simulink model "sandbox_6dof"  (R2025b)
settings: Solver=VariableStepAuto  StartTime=0.0  StopTime=10.0  RelTol=1e-3
undefined symbols (not defined in the file): AeroData, Ref_Area, rocket_length
libraries: aerolibconvert2 x3, simulink_extras x2
settings Model: Creator=jonno  LastModifiedBy=jonno

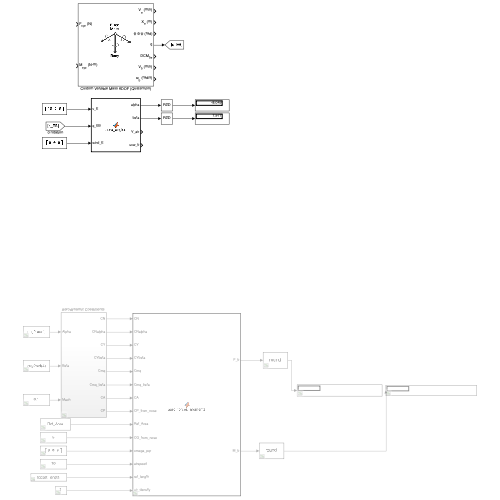
[thumbnail: Simulink's stored preview of the top-level diagram]
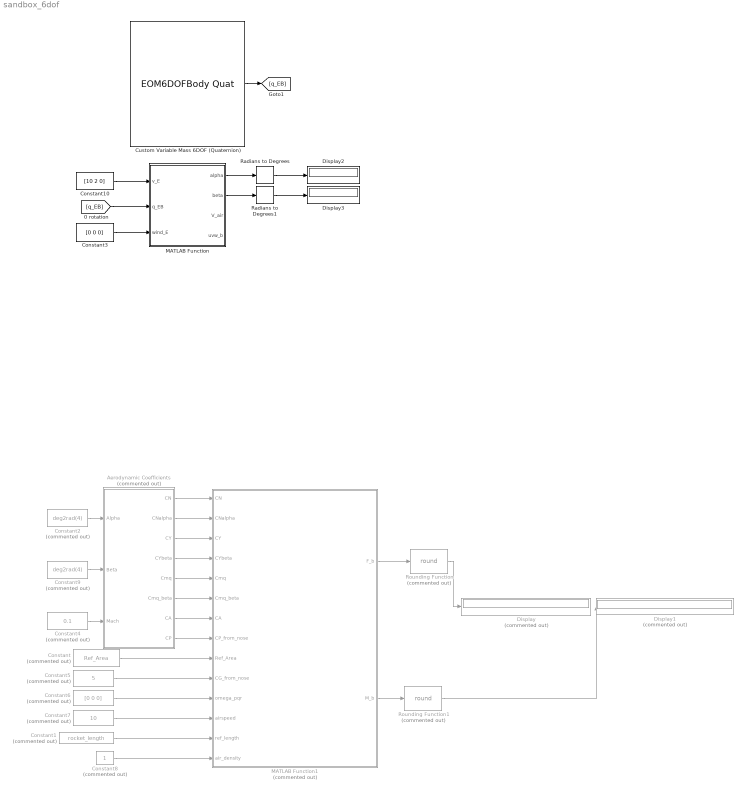
== system sandbox_6dof ==
  "Aerodynamic Coefficients " : Subsystem  Commented=on
  Constant : Constant  Commented=on  Value=Ref_Area  VectorParams1D=off
  Constant1 : Constant  Commented=on  Value=rocket_length
  Constant10 : Constant  Value=[10 2 0]
  Constant2 : Constant  Commented=on  Value=deg2rad(4)
  Constant3 : Constant  Value=[0 0 0]
  Constant4 : Constant  Commented=on  Value=0.1
  Constant5 : Constant  Commented=on  Value=5
  Constant6 : Constant  Commented=on  Value=[0 0 0]
  Constant7 : Constant  Commented=on  Value=10
  Constant8 : Constant  Commented=on
  Constant9 : Constant  Commented=on  Value=deg2rad(4)
  Custom Variable Mass 6DOF (Quaternion) : EOM6DOFBodyQuat  eul_0=[deg2rad(45) deg2rad(0) deg2rad(0)]
  Display : Display  Commented=on
  Display1 : Display  Commented=on
  Display2 : Display
  Display3 : Display
  MATLAB Function : MATLAB Function  TreatAsAtomicUnit=on
  MATLAB Function1 : MATLAB Function  Commented=on  TreatAsAtomicUnit=on
  Radians to Degrees : simulink_extras/Transformations/Radians to Degrees
  Radians to Degrees1 : simulink_extras/Transformations/Radians to Degrees
  Rounding Function : Rounding  Commented=on  Operator=round
  Rounding Function1 : Rounding  Commented=on  Operator=round
  wires:
  Custom Variable Mass 6DOF (Quaternion)/4 -> [q_EB]
  Constant10/1 -> MATLAB Function/1(v_E)
  [q_EB] -> MATLAB Function/2(q_EB)
  MATLAB Function1/1(F_b) -> Rounding Function/1
  Constant5/1 -> MATLAB Function1/10(CG_from_nose)
  Constant6/1 -> MATLAB Function1/11(omega_pqr)
  Constant8/1 -> MATLAB Function1/14(air_density)
  Constant4/1 -> "Aerodynamic Coefficients "/3(Mach)
  Constant2/1 -> "Aerodynamic Coefficients "/1(Alpha)
  "Aerodynamic Coefficients "/4(CYbeta) -> MATLAB Function1/4(CYbeta)
  "Aerodynamic Coefficients "/1(CN) -> MATLAB Function1/1(CN)
  Constant/1 -> MATLAB Function1/9(Ref_Area)
  Constant7/1 -> MATLAB Function1/12(airspeed)
  "Aerodynamic Coefficients "/8(CP) -> MATLAB Function1/8(CP_from_nose)
  "Aerodynamic Coefficients "/6(Cmq_beta) -> MATLAB Function1/6(Cmq_beta)
  "Aerodynamic Coefficients "/5(Cmq) -> MATLAB Function1/5(Cmq)
  Constant9/1 -> "Aerodynamic Coefficients "/2(Beta)
  "Aerodynamic Coefficients "/7(CA) -> MATLAB Function1/7(CA)
  "Aerodynamic Coefficients "/3(CY) -> MATLAB Function1/3(CY)
  "Aerodynamic Coefficients "/2(CNalpha) -> MATLAB Function1/2(CNalpha)
  MATLAB Function1/2(M_b) -> Rounding Function1/1
  Constant1/1 -> MATLAB Function1/13(ref_length)
  Rounding Function1/1 -> Display1/1
  Rounding Function/1 -> Display/1
  MATLAB Function/1(alpha) -> Radians to Degrees/1
  MATLAB Function/2(beta) -> Radians to Degrees1/1
  Constant3/1 -> MATLAB Function/3(wind_E)
  Radians to Degrees/1 -> Display2/1
  Radians to Degrees1/1 -> Display3/1

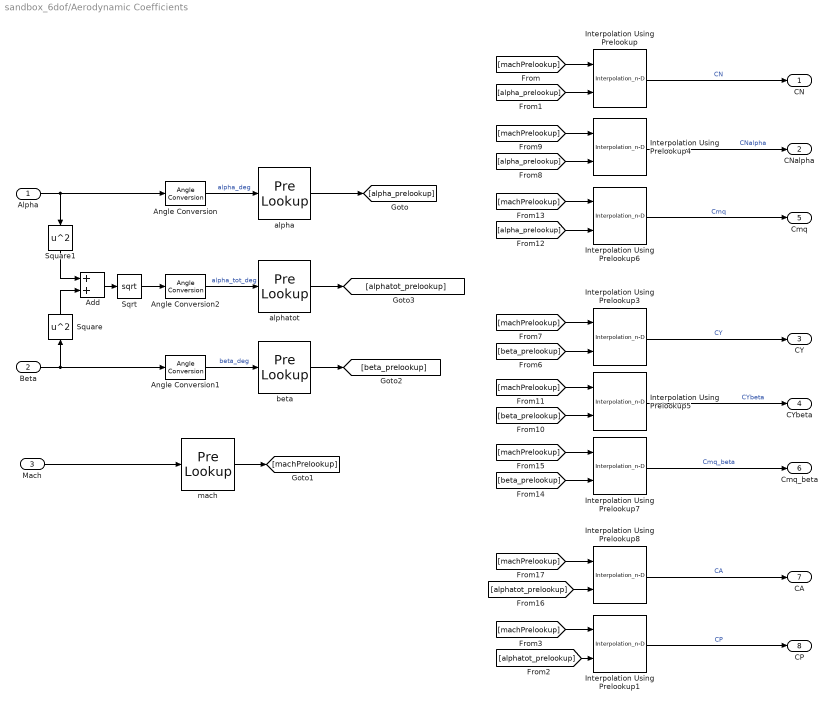
== system sandbox_6dof/Aerodynamic Coefficients  ==
  Alpha : Inport
  Beta : Inport  Port=2
  Mach : Inport  Port=3
  Add : Sum
  Angle Conversion : aerolibconvert2/Angle Conversion  IU=rad  OU=deg
  Angle Conversion1 : aerolibconvert2/Angle Conversion  IU=rad  OU=deg
  Angle Conversion2 : aerolibconvert2/Angle Conversion  IU=rad  OU=deg
  Interpolation Using Prelookup : Interpolation_n-D  Table=AeroData.Tables.CN  RequireIndexFractionAsBus=on  InternalRulePriority=Speed
      settings: InputPortMap=u0,u1
  Interpolation Using Prelookup1 : Interpolation_n-D  Table=AeroData.Tables.CP  RequireIndexFractionAsBus=on  InternalRulePriority=Speed
      settings: InputPortMap=u0,u1
  Interpolation Using Prelookup3 : Interpolation_n-D  Table=AeroData.Tables.CY  RequireIndexFractionAsBus=on  InternalRulePriority=Speed
      settings: InputPortMap=u0,u1
  Interpolation Using Prelookup4 : Interpolation_n-D  Table=AeroData.Tables.CNalpha  RequireIndexFractionAsBus=on  InternalRulePriority=Speed
      settings: InputPortMap=u0,u1
  Interpolation Using Prelookup5 : Interpolation_n-D  Table=AeroData.Tables.CYbeta  RequireIndexFractionAsBus=on  InternalRulePriority=Speed
      settings: InputPortMap=u0,u1
  Interpolation Using Prelookup6 : Interpolation_n-D  Table=AeroData.Tables.Cmq  RequireIndexFractionAsBus=on  InternalRulePriority=Speed
      settings: InputPortMap=u0,u1
  Interpolation Using Prelookup7 : Interpolation_n-D  Table=AeroData.Tables.Cmq_beta  RequireIndexFractionAsBus=on  InternalRulePriority=Speed
      settings: InputPortMap=u0,u1
  Interpolation Using Prelookup8 : Interpolation_n-D  Table=AeroData.Tables.CA  RequireIndexFractionAsBus=on  InternalRulePriority=Speed
      settings: InputPortMap=u0,u1
  Sqrt : Sqrt
  Square : Math  Operator=square
  Square1 : Math  Operator=square
  alpha : PreLookup  BreakpointsData=AeroData.Breakpoints.Alpha  OutputSelection=Index and fraction as bus  IndexSearchMethod=Evenly spaced points  UseLastBreakpoint=on
  alphatot : PreLookup  BreakpointsData=AeroData.Breakpoints.AlphaTot  OutputSelection=Index and fraction as bus  IndexSearchMethod=Evenly spaced points  UseLastBreakpoint=on
  beta : PreLookup  BreakpointsData=AeroData.Breakpoints.Beta  OutputSelection=Index and fraction as bus  IndexSearchMethod=Evenly spaced points  UseLastBreakpoint=on
  mach : PreLookup  BreakpointsData=AeroData.Breakpoints.Mach  OutputSelection=Index and fraction as bus  IndexSearchMethod=Evenly spaced points  ExtrapMethod=Linear
  CN : Outport
  CNalpha : Outport  Port=2
  CY : Outport  Port=3
  CYbeta : Outport  Port=4
  Cmq : Outport  Port=5
  Cmq_beta : Outport  Port=6
  CA : Outport  Port=7
  CP : Outport  Port=8
  wires:
  Interpolation Using Prelookup/1 -> CN/1  "CN"
  alpha/1 -> [alpha_prelookup]
  mach/1 -> [machPrelookup]
  [machPrelookup] -> Interpolation Using Prelookup/1
  [alpha_prelookup] -> Interpolation Using Prelookup/2
  Angle Conversion/1 -> alpha/1  "alpha_deg"
  Mach/1 -> mach/1
  Alpha/1 -> Square1/1, Angle Conversion/1
  Beta/1 -> Square/1, Angle Conversion1/1
  Angle Conversion1/1 -> beta/1  "beta_deg"
  beta/1 -> [beta_prelookup]
  Add/1 -> Sqrt/1
  Square1/1 -> Add/1
  Square/1 -> Add/2
  alphatot/1 -> [alphatot_prelookup]
  Angle Conversion2/1 -> alphatot/1  "alpha_tot_deg"
  Sqrt/1 -> Angle Conversion2/1
  [alpha_prelookup] -> Interpolation Using Prelookup4/2
  [machPrelookup] -> Interpolation Using Prelookup4/1
  Interpolation Using Prelookup4/1 -> CNalpha/1  "CNalpha"
  [machPrelookup] -> Interpolation Using Prelookup3/1
  [beta_prelookup] -> Interpolation Using Prelookup3/2
  Interpolation Using Prelookup3/1 -> CY/1  "CY"
  [machPrelookup] -> Interpolation Using Prelookup5/1
  Interpolation Using Prelookup5/1 -> CYbeta/1  "CYbeta"
  [beta_prelookup] -> Interpolation Using Prelookup5/2
  [machPrelookup] -> Interpolation Using Prelookup6/1
  [alpha_prelookup] -> Interpolation Using Prelookup6/2
  Interpolation Using Prelookup6/1 -> Cmq/1  "Cmq"
  [machPrelookup] -> Interpolation Using Prelookup7/1
  Interpolation Using Prelookup7/1 -> Cmq_beta/1  "Cmq_beta"
  [beta_prelookup] -> Interpolation Using Prelookup7/2
  [machPrelookup] -> Interpolation Using Prelookup8/1
  Interpolation Using Prelookup8/1 -> CA/1  "CA"
  [alphatot_prelookup] -> Interpolation Using Prelookup8/2
  Interpolation Using Prelookup1/1 -> CP/1  "CP"
  [alphatot_prelookup] -> Interpolation Using Prelookup1/2
  [machPrelookup] -> Interpolation Using Prelookup1/1

== matlab function sandbox_6dof/MATLAB Function ==
  data: v_E input; alpha output; q_EB input; wind_E input; beta output; V_air output; uvw_b output
function [alpha, beta, V_air, uvw_b] = aero_angles(v_E, q_EB, wind_E)
% Aerodynamic angles from Earth velocity, quaternion (Earth->Body), and wind.
% Convention: positive beta = wind from the RIGHT (opposite thesis sign)
% Units: radians, m/s

% -- Parameters
VEL_EPS = 1e-6;

% -- Quaternion normalization (scalar-first)
q = q_EB(:).';
q = q / max(norm(q), eps);

% -- Rotation Earth->Body (passive)
R_BE = quat2dcm(q);  % Aerospace Toolbox, scalar-first

% -- Relative air-velocity in body axes
v_rel_E = v_E(:) - wind_E(:);
uvw_b   = R_BE * v_rel_E;
u = uvw_b(1); v = uvw_b(2); w = uvw_b(3);
V_air = norm(uvw_b);

% -- Handle zero/near-zero airspeed
if V_air < VEL_EPS
    alpha = 0.0;
    beta  = 0.0;
    uvw_b = [0;0;0];
    V_air = 0.0;
    return
end

% -- Aerodynamic angles (robust)
alpha = atan2(w, u);
beta  = asin( max(-1, min(1, v / V_air)) );  % FLIP SIGN for "positive beta = wind from right"
end

== matlab function sandbox_6dof/MATLAB Function1 ==
  data: CN input; F_b output; CNalpha input; CY input; CYbeta input; Cmq input; Cmq_beta input; CA input; CP_from_nose input; Ref_Area input; CG_from_nose input; omega_pqr input; airspeed input; ref_length input; air_density input; M_b output
function [F_b, M_b] = aero_forces_moments( ...
    CN, CNalpha, CY, CYbeta, Cmq, Cmq_beta, CA, CP_from_nose, ...
    Ref_Area, CG_from_nose, omega_pqr, airspeed, ref_length, air_density)
% Aero forces and moments (body axes), with beta convention:
%   Positive beta = wind from the right
% Inputs:
%   CN, CY, CA             : force coefficients
%   CNalpha, CYbeta        : slopes (reserved)
%   Cmq, Cmq_beta          : damping (pitch/yaw), lumped
%   CP_from_nose, CG_from_nose : [m]
%   Ref_Area               : [m^2]
%   ref_length             : [m]
%   omega_pqr              : [rad/s] [p; q; r]
%   airspeed               : [m/s]
%   air_density            : [kg/m^3]
% Outputs:
%   F_b = [Fx; Fy; Fz], M_b = [Mx; My; Mz]

% --- Precompute
S  = Ref_Area;
d  = ref_length;
V  = max(airspeed, 1e-6);
q_dyn = 0.5 * air_density * V * V;
Lcp = CP_from_nose - CG_from_nose;

% Body rates
p = omega_pqr(1);
q = omega_pqr(2);
r = omega_pqr(3);

% --- Adjust lateral force for beta sign convention (positive beta = wind from right)
CY_eff = -CY;

% --- Forces (x forward, y right, z down)
Fx = - q_dyn * S * CA;
Fy =   q_dyn * S * CY_eff;
Fz = - q_dyn * S * CN;

% --- Static moments from CP lever arm
M_stat_x = 0.0;
M_stat_y = - q_dyn * S * CN     * Lcp;
M_stat_z = - q_dyn * S * CY_eff * Lcp;

% --- Rate damping with d/(2V) (Cmq and Cmq_beta are negative for damping, keep as-is)
scale = d / (2.0 * V);
M_damp_y = q_dyn * S * d * ( scale * Cmq      * q );
M_damp_z = q_dyn * S * d * ( scale * Cmq_beta * r );

% --- Totals
Mx = M_stat_x;
My = M_stat_y + M_damp_y;
Mz = M_stat_z + M_damp_z;

F_b = [Fx; Fy; Fz];
M_b = [Mx; My; Mz];
end
